simulink model "vehicle_3dof"  (R2014a)
settings: Solver=ode45  StartTime=0.0  StopTime=10.0  RelTol=1e-3
values from neighbouring files (symbols this model uses):
  g = 9.81    [ThreeDOFVehicleModel.m]
  h = 0.4    [ThreeDOFVehicleModel.m]
  Ix = 614    [ThreeDOFVehicleModel.m]
  Iz = 2488    [ThreeDOFVehicleModel.m]
  ms = 1592    [ThreeDOFVehicleModel.m]
undefined symbols (not defined in the file or in its folder): Cf, Cfif, Cfir, H, hs, Kfif, Kfir, lf, lr, mt, tw, v0x
settings Model: Creator=Mac  LastModifiedBy=57371

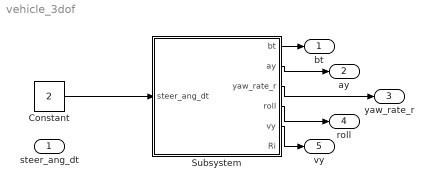
== system vehicle_3dof ==
  steer_ang_dt : Inport
  Constant : Constant  Value=2
  Subsystem : Subsystem
  bt : Outport
  ay : Outport  Port=2
  yaw_rate_r : Outport  Port=3
  roll : Outport  Port=4
  vy : Outport  Port=5
  wires:
  Constant/1 -> Subsystem/1(steer_ang_dt)
  Subsystem/1(bt) -> bt/1
  Subsystem/2(ay) -> ay/1
  Subsystem/3(yaw_rate_r) -> yaw_rate_r/1
  Subsystem/4(roll) -> roll/1
  Subsystem/5(vy) -> vy/1

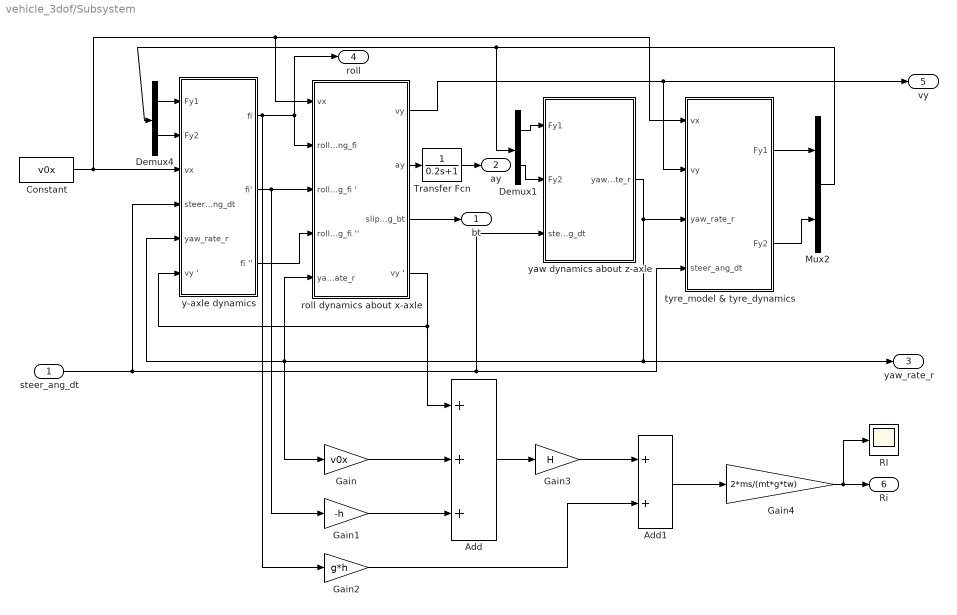
== system vehicle_3dof/Subsystem ==
  steer_ang_dt : Inport
  Add : Sum  Inputs=+++
  Add1 : Sum
  Constant : Constant  Value=v0x
  Demux1 : Demux  Outputs=2
  Demux4 : Demux  Outputs=2
  Gain : Gain  Gain=v0x
  Gain1 : Gain  Gain=-h
  Gain2 : Gain  Gain=g*h
  Gain3 : Gain  Gain=H
  Gain4 : Gain  Gain=2*ms/(mt*g*tw)
  Mux2 : Mux  Inputs=2
  RI : Scope
  Transfer Fcn : TransferFcn  Denominator=[0.2 1]
  roll dynamics about x-axle : Subsystem
  tyre_model & tyre_dynamics : Subsystem
  y-axle dynamics : Subsystem
  yaw dynamics about z-axle : Subsystem
  bt : Outport
  ay : Outport  Port=2
  yaw_rate_r : Outport  Port=3
  roll : Outport  Port=4
  vy : Outport  Port=5
  Ri : Outport  Port=6
  wires:
  Demux4/1 -> y-axle dynamics/1(Fy1)
  Transfer Fcn/1 -> ay/1
  Demux4/2 -> y-axle dynamics/2(Fy2)
  Demux1/2 -> yaw dynamics about z-axle/2(Fy2)
  tyre_model & tyre_dynamics/2(Fy2) -> Mux2/2
  roll dynamics about x-axle/2(ay) -> Transfer Fcn/1
  tyre_model & tyre_dynamics/1(Fy1) -> Mux2/1
  y-axle dynamics/3(fi '') -> roll dynamics about x-axle/4(roll_ang_fi '')
  yaw dynamics about z-axle/1("yaw_rate_r ") -> tyre_model & tyre_dynamics/3(yaw_rate_r), yaw_rate_r/1, Gain/1, roll dynamics about x-axle/5(yaw_rate_r), y-axle dynamics/5(yaw_rate_r)
  Demux1/1 -> yaw dynamics about z-axle/1(Fy1)
  Constant/1 -> y-axle dynamics/3(vx), tyre_model & tyre_dynamics/1(vx), roll dynamics about x-axle/1(vx)
  Mux2/1 -> Demux1/1, Demux4/1
  roll dynamics about x-axle/4(vy ') -> Add/1, y-axle dynamics/6(vy ')
  roll dynamics about x-axle/3(slip_ang_bt) -> bt/1
  y-axle dynamics/2(fi') -> roll dynamics about x-axle/3(roll_ang_fi '), Gain1/1
  steer_ang_dt/1 -> yaw dynamics about z-axle/3(steer_ang_dt), tyre_model & tyre_dynamics/4(steer_ang_dt), y-axle dynamics/4(steer_ang_dt)
  roll dynamics about x-axle/1(vy) -> vy/1, tyre_model & tyre_dynamics/2(vy)
  y-axle dynamics/1(fi) -> roll/1, roll dynamics about x-axle/2("roll_ang_fi "), Gain2/1
  Gain/1 -> Add/2
  Gain1/1 -> Add/3
  Add/1 -> Gain3/1
  Gain3/1 -> Add1/1
  Gain2/1 -> Add1/2
  Add1/1 -> Gain4/1
  Gain4/1 -> RI/1, Ri/1

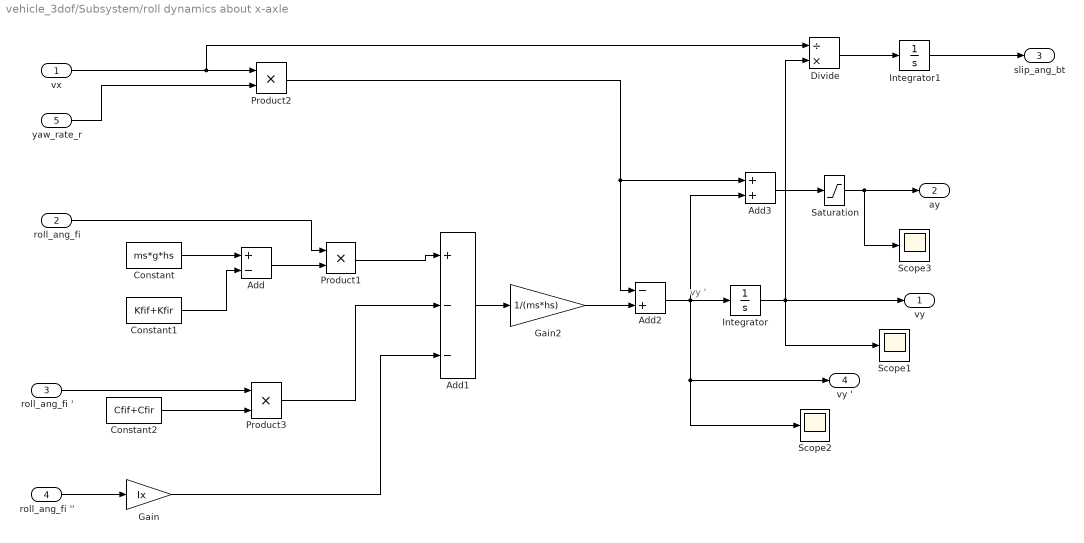
== system vehicle_3dof/Subsystem/roll dynamics about x-axle ==
  note: vy '
  vx : Inport
  "roll_ang_fi " : Inport  Port=2
  roll_ang_fi ' : Inport  Port=3
  roll_ang_fi '' : Inport  Port=4
  yaw_rate_r : Inport  Port=5
  Add : Sum  Inputs=+-
  Add1 : Sum  Inputs=+--
  Add2 : Sum  Inputs=-+
  Add3 : Sum
  Constant : Constant  Value=ms*g*hs
  Constant1 : Constant  Value=Kfif+Kfir
  Constant2 : Constant  Value=Cfif+Cfir
  Divide : Product  Inputs=/*
  Gain : Gain  Gain=Ix
  Gain2 : Gain  Gain=1/(ms*hs)
  Integrator : Integrator
  Integrator1 : Integrator
  Product1 : Product  RndMeth=Zero
  Product2 : Product  RndMeth=Zero
  Product3 : Product  RndMeth=Zero
  Saturation : Saturate  UpperLimit=9.8  LowerLimit=-9.8
  Scope1 : Scope
      settings: TimeRange=6  YMin=-0.1  YMax=0  SaveName=ScopeData15
  Scope2 : Scope
      settings: TimeRange=6  YMin=-0.1  YMax=0  SaveName=ScopeData16
  Scope3 : Scope
      settings: TimeRange=6  YMin=-0.1  YMax=0  SaveName=ScopeData17
  vy : Outport
  ay : Outport  Port=2
  slip_ang_bt : Outport  Port=3
  vy ' : Outport  Port=4
  wires:
  Constant/1 -> Add/1
  Constant1/1 -> Add/2
  Product2/1 -> Add2/1, Add3/1
  Add/1 -> Product1/2
  "roll_ang_fi "/1 -> Product1/1
  roll_ang_fi '/1 -> Product3/1
  Constant2/1 -> Product3/2
  Product1/1 -> Add1/1
  Product3/1 -> Add1/2
  roll_ang_fi ''/1 -> Gain/1
  Gain/1 -> Add1/3
  Add1/1 -> Gain2/1
  vx/1 -> Product2/1, Divide/1
  yaw_rate_r/1 -> Product2/2
  Gain2/1 -> Add2/2
  Add2/1 -> Integrator/1, Add3/2, vy '/1, Scope2/1
  Integrator/1 -> Divide/2, vy/1, Scope1/1
  Add3/1 -> Saturation/1
  Saturation/1 -> ay/1, Scope3/1
  Integrator1/1 -> slip_ang_bt/1
  Divide/1 -> Integrator1/1

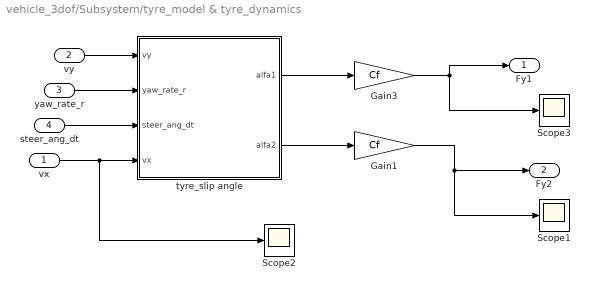
== system vehicle_3dof/Subsystem/tyre_model & tyre_dynamics ==
  vx : Inport
  vy : Inport  Port=2
  yaw_rate_r : Inport  Port=3
  steer_ang_dt : Inport  Port=4
  Gain1 : Gain  Gain=Cf
  Gain3 : Gain  Gain=Cf
  Scope1 : Scope
      settings: SaveName=ScopeData3
  Scope2 : Scope
      settings: SaveName=ScopeData5
  Scope3 : Scope
      settings: SaveName=ScopeData8
  "tyre_slip angle " : Subsystem
  Fy1 : Outport
  Fy2 : Outport  Port=2
  wires:
  vx/1 -> Scope2/1, "tyre_slip angle "/4(vx)
  vy/1 -> "tyre_slip angle "/1(vy)
  yaw_rate_r/1 -> "tyre_slip angle "/2(yaw_rate_r)
  steer_ang_dt/1 -> "tyre_slip angle "/3(steer_ang_dt)
  Gain3/1 -> Fy1/1, Scope3/1
  "tyre_slip angle "/1(alfa1) -> Gain3/1
  "tyre_slip angle "/2(alfa2) -> Gain1/1
  Gain1/1 -> Fy2/1, Scope1/1

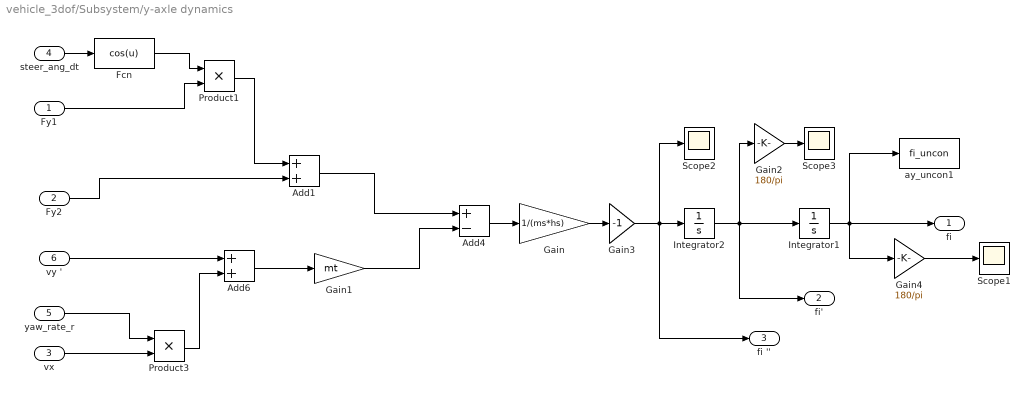
== system vehicle_3dof/Subsystem/y-axle dynamics ==
  Fy1 : Inport
  Fy2 : Inport  Port=2
  vx : Inport  Port=3
  steer_ang_dt : Inport  Port=4
  yaw_rate_r : Inport  Port=5
  vy ' : Inport  Port=6
  Add1 : Sum
  Add4 : Sum  Inputs=+-
  Add6 : Sum
  Fcn : Fcn  Expr=cos(u)
  Gain : Gain  Gain=1/(ms*hs)
  Gain1 : Gain  Gain=mt
  Gain2 : Gain  Gain=180/pi
  Gain3 : Gain  Gain=-1
  Gain4 : Gain  Gain=180/pi
  Integrator1 : Integrator
  Integrator2 : Integrator
  Product1 : Product  RndMeth=Zero
  Product3 : Product  RndMeth=Zero
  Scope1 : Scope
      settings: TimeRange=6  YMin=-0.1  YMax=0  SaveName=ScopeData10
  Scope2 : Scope
      settings: TimeRange=6  YMin=-0.1  YMax=0  SaveName=ScopeData13
  Scope3 : Scope
      settings: TimeRange=6  YMin=-0.1  YMax=0  SaveName=ScopeData14
  ay_uncon1 : ToWorkspace  VariableName=fi_uncon  SampleTime=-1
  fi : Outport
  fi' : Outport  Port=2
  fi '' : Outport  Port=3
  wires:
  steer_ang_dt/1 -> Fcn/1
  Fy1/1 -> Product1/2
  yaw_rate_r/1 -> Product3/1
  Add4/1 -> Gain/1
  vx/1 -> Product3/2
  Fy2/1 -> Add1/2
  Gain/1 -> Gain3/1
  Integrator2/1 -> fi'/1, Gain2/1, Integrator1/1
  Integrator1/1 -> fi/1, ay_uncon1/1, Gain4/1
  vy '/1 -> Add6/1
  Product3/1 -> Add6/2
  Gain1/1 -> Add4/2
  Add6/1 -> Gain1/1
  Fcn/1 -> Product1/1
  Product1/1 -> Add1/1
  Add1/1 -> Add4/1
  Gain2/1 -> Scope3/1
  Gain3/1 -> Integrator2/1, fi ''/1, Scope2/1
  Gain4/1 -> Scope1/1

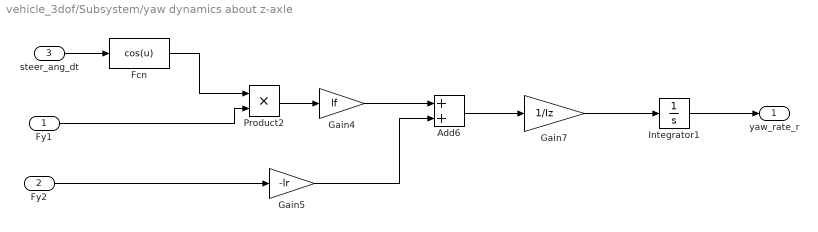
== system vehicle_3dof/Subsystem/yaw dynamics about z-axle ==
  Fy1 : Inport
  Fy2 : Inport  Port=2
  steer_ang_dt : Inport  Port=3
  Add6 : Sum
  Fcn : Fcn  Expr=cos(u)
  Gain4 : Gain  Gain=lf
  Gain5 : Gain  Gain=-lr
  Gain7 : Gain  Gain=1/Iz
  Integrator1 : Integrator
  Product2 : Product  RndMeth=Zero
  "yaw_rate_r " : Outport
  wires:
  steer_ang_dt/1 -> Fcn/1
  Fy1/1 -> Product2/2
  Product2/1 -> Gain4/1
  Fy2/1 -> Gain5/1
  Gain5/1 -> Add6/2
  Gain7/1 -> Integrator1/1
  Integrator1/1 -> "yaw_rate_r "/1
  Fcn/1 -> Product2/1
  Gain4/1 -> Add6/1
  Add6/1 -> Gain7/1

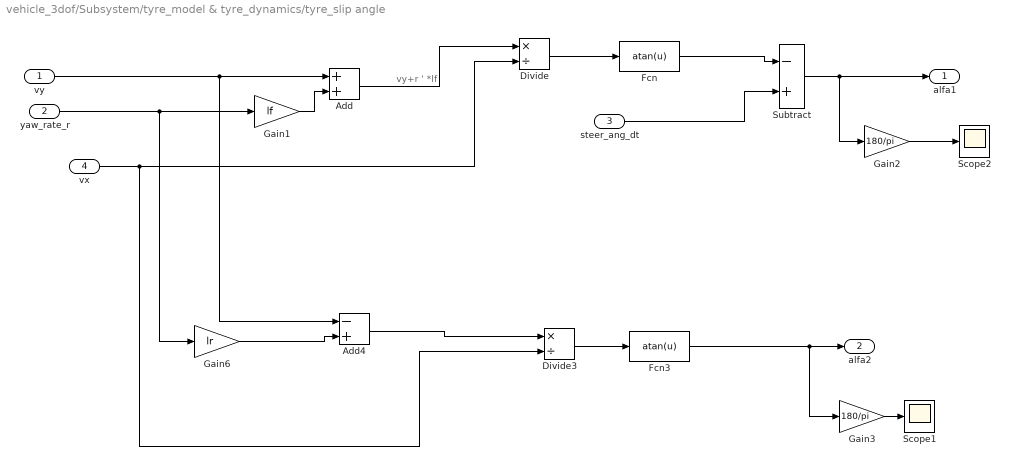
== system vehicle_3dof/Subsystem/tyre_model & tyre_dynamics/tyre_slip angle  ==
  note: vy+r ' *lf
  vy : Inport
  yaw_rate_r : Inport  Port=2
  steer_ang_dt : Inport  Port=3
  vx : Inport  Port=4
  Add : Sum
  Add4 : Sum  Inputs=-+
  Divide : Product  Inputs=*/
  Divide3 : Product  Inputs=*/
  Fcn : Fcn  Expr=atan(u)
  Fcn3 : Fcn  Expr=atan(u)
  Gain1 : Gain  Gain=lf
  Gain2 : Gain  Gain=180/pi
  Gain3 : Gain  Gain=180/pi
  Gain6 : Gain  Gain=lr
  Scope1 : Scope
      settings: SaveName=ScopeData11
  Scope2 : Scope
      settings: SaveName=ScopeData12
  Subtract : Sum  Inputs=-+
  alfa1 : Outport
  alfa2 : Outport  Port=2
  wires:
  vy/1 -> Add/1, Add4/1
  Fcn/1 -> Subtract/1
  yaw_rate_r/1 -> Gain1/1, Gain6/1
  Gain1/1 -> Add/2
  Add/1 -> Divide/1
  Divide/1 -> Fcn/1
  steer_ang_dt/1 -> Subtract/2
  Gain6/1 -> Add4/2
  Divide3/1 -> Fcn3/1
  Fcn3/1 -> alfa2/1, Gain3/1
  Add4/1 -> Divide3/1
  vx/1 -> Divide/2, Divide3/2
  Subtract/1 -> alfa1/1, Gain2/1
  Gain2/1 -> Scope2/1
  Gain3/1 -> Scope1/1
